simulink model "pi_transmitter"  (R2017a)
settings: Solver=FixedStepDiscrete  StartTime=0.0  StopTime=5.0  FixedStep=1/40  RelTol=1e-3  EnableMultiTasking=on
undefined symbols (not defined in the file or in its folder): Green, led0
libraries: embdlinuxlib x1, raspberrypilib x1
settings Model: SimulationMode=external  Creator=Vincent  LastModifiedBy=Vincent
settings SolverCC: PositivePriorityOrder=on
settings OptimizationCC: PassReuseOutputArgsThreshold=0  MaxStackSize=64
settings DebuggingCC: ParameterTunabilityLossMsg=error
settings HardwareCC: ProdBitPerPointer=32  ProdBitPerSizeT=32  ProdBitPerPtrDiffT=32  ProdLargestAtomicInteger=Long  ProdLargestAtomicFloat=Double  ProdWordSize=32  ProdHWDeviceType=ARM Compatible->ARM Cortex  UseEmbeddedCoderFeatures=off
settings SFSimCC: MATLABDynamicMemAlloc=off
settings RTWCC: SystemTargetFile=ert.tlc  HardwareBoard=Raspberry Pi  TLCOptions="-aInlineSetEventsForThisBaseRateFcn=TLC_FALSE -aSuppressMultiTaskScheduler=TLC_FALSE  -aRateBasedStepFcn=0"  TemplateMakefile=ert_default_tmf  Description=Embedded Coder  GenerateReport=on  Toolchain=GNU GCC Raspberry Pi  LaunchReport=on
settings CodeAppCC: ForceParamTrailComments=on  OperatorAnnotations=on  MATLABSourceComments=on
settings ERTTargetCC: ERTCustomFileBanners=off  SupportContinuousTime=on  SupportNonInlinedSFcns=on  RemoveResetFunc=off  SupportVariableSizeSignals=on  ModelStepFunctionPrototypeControlCompliant=off

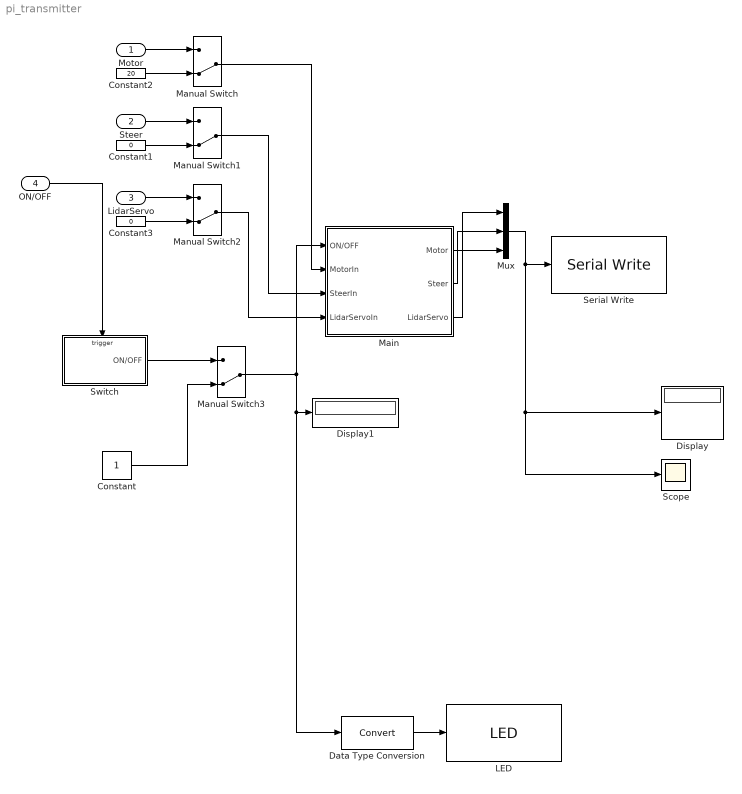
== system pi_transmitter ==
  Motor : Inport
  Steer : Inport  Port=2
  LidarServo : Inport  Port=3
  ON/OFF : Inport  Port=4
  Constant : Constant
  Constant1 : Constant  Value=0
  Constant2 : Constant  Value=20
  Constant3 : Constant  Value=0
  Data Type Conversion : DataTypeConversion
  Display : Display
  Display1 : Display
  LED : embdlinuxlib/LED  board=Model B+  led=led0 (Green)  blockPlatform=Raspberry Pi
  Main : Subsystem  TreatAsAtomicUnit=on
  Manual Switch{,1..3} (4 alike) : ManualSwitch  CurrentSetting=0
  Mux : Mux  Inputs=3
  Scope : Scope
  Serial Write : raspberrypilib/Serial Write  board=Pi 3 Model B  SCIModule_=/dev/ttyS0  Baudrate_=9600  Parity=None  StopBits_=1  HardwareFlowControl=None  ByteOrder=LittleEndian  OutputStatus=off  blockPlatform=RaspberryPi
      settings: SourceProductName=Simulink Support Package for Raspberry Pi Hardware  SourceProductBaseCode=RASPPI
  Switch : Subsystem  TreatAsAtomicUnit=on
  wires:
  Main/3(LidarServo) -> Mux/1
  Main/1(Motor) -> Mux/3
  Main/2(Steer) -> Mux/2
  Manual Switch3/1 -> Main/1(ON/OFF), Display1/1, Data Type Conversion/1
  Mux/1 -> Serial Write/1, Scope/1, Display/1
  ON/OFF/1 -> Switch/Trigger
  Switch/1(ON/OFF) -> Manual Switch3/1
  Data Type Conversion/1 -> LED/1
  Constant/1 -> Manual Switch3/2
  Motor/1 -> Manual Switch/1
  Constant2/1 -> Manual Switch/2
  Manual Switch/1 -> Main/2(MotorIn)
  Steer/1 -> Manual Switch1/1
  Manual Switch1/1 -> Main/3("SteerIn ")
  Constant1/1 -> Manual Switch1/2
  LidarServo/1 -> Manual Switch2/1
  Constant3/1 -> Manual Switch2/2
  Manual Switch2/1 -> Main/4(LidarServoIn)

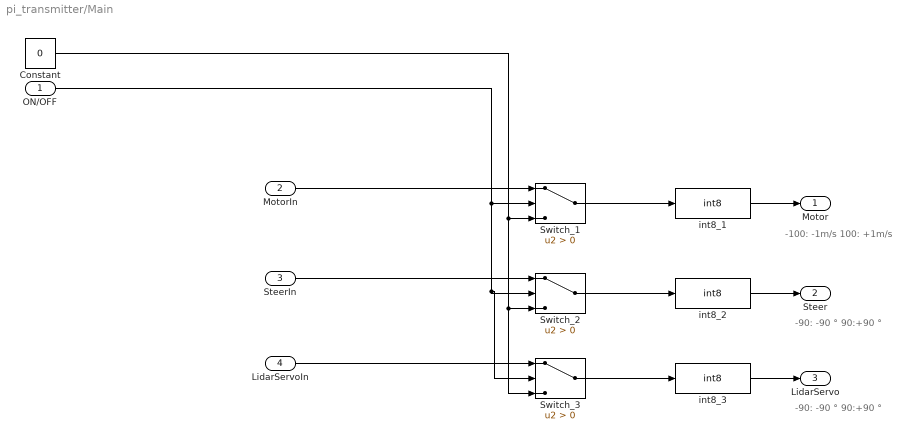
== system pi_transmitter/Main ==
  note: -100: -1m/s
      | 100: +1m/s
  note: -90: -90 °
      | 90:+90 °
  note: -90: -90 °
      | 90:+90 °
  ON/OFF : Inport
  MotorIn : Inport  Port=2
  "SteerIn " : Inport  Port=3
  LidarServoIn : Inport  Port=4
  Constant : Constant  Value=0
  Switch_1 : Switch  Criteria=u2 > Threshold
  Switch_2 : Switch  Criteria=u2 > Threshold
  Switch_3 : Switch  Criteria=u2 > Threshold
  int8_1 : DataTypeConversion  OutDataTypeStr=int8
  int8_2 : DataTypeConversion  OutDataTypeStr=int8
  int8_3 : DataTypeConversion  OutDataTypeStr=int8
  Motor : Outport
  Steer : Outport  Port=2
  LidarServo : Outport  Port=3
  wires:
  int8_2/1 -> Steer/1
  int8_3/1 -> LidarServo/1
  int8_1/1 -> Motor/1
  Switch_2/1 -> int8_2/1
  Switch_3/1 -> int8_3/1
  "SteerIn "/1 -> Switch_2/1
  ON/OFF/1 -> Switch_3/2, Switch_2/2, Switch_1/2
  Constant/1 -> Switch_3/3, Switch_2/3, Switch_1/3
  Switch_1/1 -> int8_1/1
  LidarServoIn/1 -> Switch_3/1
  MotorIn/1 -> Switch_1/1

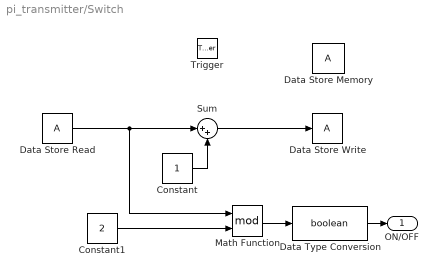
== system pi_transmitter/Switch ==
  Trigger : TriggerPort  VariantControl=Variant
  Constant : Constant
  Constant1 : Constant  Value=2
  Data Store Memory : DataStoreMemory  ReadBeforeWriteMsg=warning  WriteAfterWriteMsg=warning  WriteAfterReadMsg=warning  ShowAdditionalParam=off
  Data Store Read : DataStoreRead
  Data Store Write : DataStoreWrite
  Data Type Conversion : DataTypeConversion  OutDataTypeStr=boolean
  Math Function : Math  Operator=mod  SaturateOnIntegerOverflow=on
  Sum : Sum  Inputs=|++
  ON/OFF : Outport
  wires:
  Sum/1 -> Data Store Write/1
  Data Store Read/1 -> Math Function/1, Sum/1
  Constant/1 -> Sum/2
  Constant1/1 -> Math Function/2
  Math Function/1 -> Data Type Conversion/1
  Data Type Conversion/1 -> ON/OFF/1
